simulink model "my_rfb_receiver_0"  (R2014b)
settings: Solver=FixedStepDiscrete  SolverMode=SingleTasking  StartTime=0.0  StopTime=inf  RelTol=1e-3
PostLoadFcn:
  | noiseVec = [2 3.5 5 25];
  | gainVec = 10.0.^(0.05*[-2 30 -6 35]);
  | oip3Vec = [100 100 100 100];
  | EbNo = 13; % dB
  | M = 4; % bits per symbol
  | maxerr = 100;
  | maxbits = 1e8;
  | N = 8;  % Upsampling factor
  | rrc_delay = 4; % symbols
libraries: commutil2 x2, commfilt2 x2, commdigbbndam3 x2, commchan3 x1, commsink2 x1, commrandsrc2 x1
settings Model: FPTRunName=Active  Creator=The MathWorks Inc.  LastModifiedBy=Ben
settings DataIOCC: SignalLoggingSaveFormat=ModelDataLogs  SaveOutput=off  SaveTime=off  SignalLoggingName=sigsOut
settings OptimizationCC: ExpressionDepthLimit=2147483647  InitFltsAndDblsToZero=on  EfficientMapNaN2IntZero=off
settings DebuggingCC: SaveWithParameterizedLinksMsg=none  UnderspecifiedInitializationDetection=Classic  MergeDetectMultiDrivingBlocksExec=none  CheckExecutionContextPreStartOutputMsg=on  CheckExecutionContextRuntimeOutputMsg=on  SignalResolutionControl=TryResolveAllWithWarning  SolverPrmCheckMsg=none  InheritedTsInSrcMsg=none  MultiTaskDSMMsg=warning  MultiTaskCondExecSysMsg=none  SigSpecEnsureSampleTimeMsg=none  FcnCallInpInsideContextMsg=UseLocalSettings  StateNameClashWarn=warning  StrictBusMsg=None
settings HardwareCC: ProdHWDeviceType=Specified
settings ModelReferenceCC: UpdateModelReferenceTargets=IfOutOfDate
settings RTWCC: IncludeERTFirstTime=on
settings GRTTargetCC: TargetFcnLib=ansi_tfl_tmw.mat  CombineOutputUpdateFcns=off  GRTInterface=on

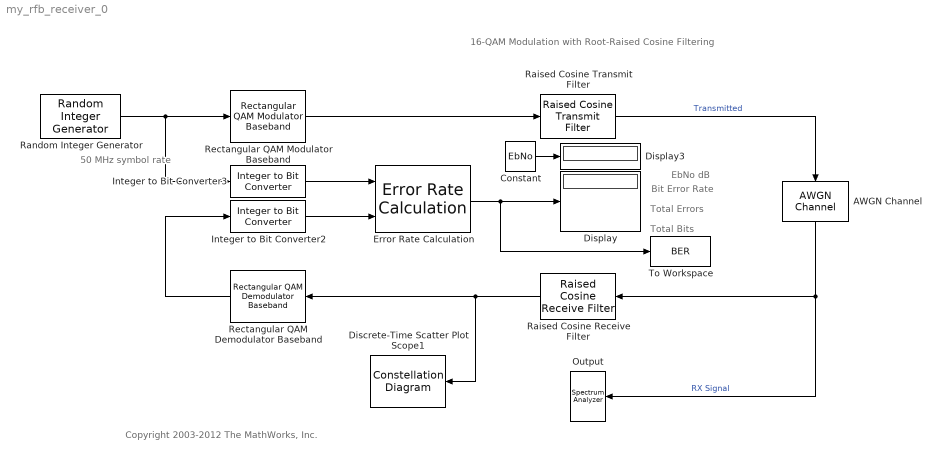
== system my_rfb_receiver_0 ==
  note: 50 MHz symbol rate
  note: 16-QAM Modulation
      | with Root-Raised Cosine Filtering
  note: Bit Error Rate
  note: Total Errors
  note: Total Bits
  note: EbNo dB
  note: Copyright 2003-2012 The MathWorks, Inc.
  AWGN Channel : commchan3/AWGN Channel  InputProcessing=Columns as channels (frame based)  seed=97  noiseMode="Signal to noise ratio  (Eb/No)"  EbNodB=EbNo  EsNodB=EbNo + 10*log10(M)  SNRdB=EbNo + 10*log10(M) - 10*log10(N)  bitsPerSym=M  Ps=1  Tsym=1/50e6  variance=10^(-EbNo/20)
  Constant : Constant  Value=EbNo
  Discrete-Time Scatter Plot Scope1 : ConstellationDiagram  Tag=ScatterPlot
  Display : Display
  Display3 : Display
  Error Rate Calculation : commsink2/Error Rate Calculation  N=2*rrc_delay*M  st_delay=2*rrc_delay*M*1024  cp_mode=Entire frame  subframe=[]  PMode=Port  WsName=QAM_BER  RsMode2=off  stop=on  numErr=maxerr  maxBits=maxbits
  Integer to Bit Converter2 : commutil2/Integer to Bit Converter  nbits=M  signedInputValues=Unsigned  bitOrder=MSB first  outDtype=Inherit via internal rule
  Integer to Bit Converter3 : commutil2/Integer to Bit Converter  nbits=M  signedInputValues=Unsigned  bitOrder=MSB first  outDtype=Inherit via internal rule
  Output : SpectrumAnalyzer
  Raised Cosine Receive Filter : commfilt2/Raised Cosine Receive Filter  filtType=Square root  N=N  filtSpan=2*(rrc_delay)  currentFiltSpan=2*(rrc_delay)  D=(2*(rrc_delay))/2  R=0.2  sampMode=Mute  saveAsFlag=0  rateMode=Downsampling  downFactor=N  downOffset=0  framing=Enforce single-rate processing  InputProcessing=Columns as channels (frame based)  checkGain=User-specified  filterGain=sqrt(1/N)  checkCoeff=off  variableName=rcRxFilt  launchFVT=off  roundingMode=Floor  overflowMode=off
  Raised Cosine Transmit Filter : commfilt2/Raised Cosine Transmit Filter  filtType=Square root  filtSpan=2*(rrc_delay)  currentFiltSpan=2*(rrc_delay)  D=(2*(rrc_delay))/2  R=0.2  sampMode=Mute  saveAsFlag=0  N=N  framing=Enforce single-rate processing  InputProcessing=Columns as channels (frame based)  checkGain=User-specified  filterGain=sqrt(N)  checkCoeff=off  variableName=rcTxFilt  launchFVT=off  roundingMode=Floor  overflowMode=off
  Random Integer Generator : commrandsrc2/Random Integer Generator  mul=2^M  seed=37  Ts=2e-8  frameBased=on  sampPerFrame=1024  orient=off  outDataType=double
  Rectangular QAM Demodulator Baseband : commdigbbndam3/Rectangular QAM Demodulator Baseband  M=2^M  PowType=Average Power  MinDist=sqrt(2)/(sqrt(2^M)-1)  AvgPow=1  PeakPow=2  Ph=0  Dec=Gray  Mapping=[0:15]  OutType=Integer  DecType=Hard decision  VarSource=Dialog  Variance=1  outDtype1=double  outDtype2=double  derotateFactorWordLen=16  denormFactorWordLen=16  prodOutWordLen=32  prodOutRoundingMode=Floor  prodOutOverflowMode=Wrap  sumWordLen=32
  Rectangular QAM Modulator Baseband : commdigbbndam3/Rectangular QAM Modulator Baseband  M=2^M  InType=Integer  Enc=Gray  Mapping=[0:15]  PowType=Average Power  MinDist=sqrt(2)/(sqrt(2^M)-1)  AvgPow=1  PeakPow=2  Ph=0  outDtype=double  outWordLen=16  outUDDataType=sfix(16)  outFracLenMode=Best precision  outFracLen=15
  To Workspace : ToWorkspace  VariableName=BER  SampleTime=-1
      settings: MaxDataPoints=1
  wires:
  Random Integer Generator/1 -> Rectangular QAM Modulator Baseband/1, Integer to Bit Converter3/1
  Raised Cosine Transmit Filter/1 -> AWGN Channel/1  "Transmitted"
  Raised Cosine Receive Filter/1 -> Rectangular QAM Demodulator Baseband/1, Discrete-Time Scatter Plot Scope1/1
  AWGN Channel/1 -> Raised Cosine Receive Filter/1, Output/1  "RX Signal"
  Integer to Bit Converter3/1 -> Error Rate Calculation/1
  Integer to Bit Converter2/1 -> Error Rate Calculation/2
  Error Rate Calculation/1 -> Display/1, To Workspace/1
  Rectangular QAM Demodulator Baseband/1 -> Integer to Bit Converter2/1
  Rectangular QAM Modulator Baseband/1 -> Raised Cosine Transmit Filter/1
  Constant/1 -> Display3/1
